simulink model "Baro"  (R2021a)
settings: Solver=VariableStepAuto  StartTime=0.0  StopTime=10.0  RelTol=1e-3
undefined symbols (not defined in the file or in its folder): Sensor_err
libraries: dspsrcs4 x1
settings Model: Creator=mojta  LastModifiedBy=mojta

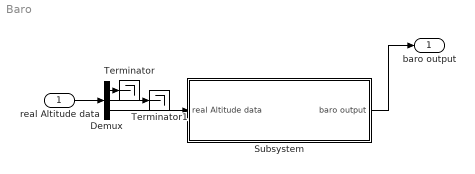
== system Baro ==
  real Altitude data : Inport
  Demux : Demux  Outputs=3
  Subsystem : Subsystem
  Terminator : Terminator
  Terminator1 : Terminator
  baro output : Outport
  wires:
  Demux/3 -> Subsystem/1(real Altitude data)
  Subsystem/1(baro output) -> baro output/1
  real Altitude data/1 -> Demux/1
  Demux/1 -> Terminator/1
  Demux/2 -> Terminator1/1

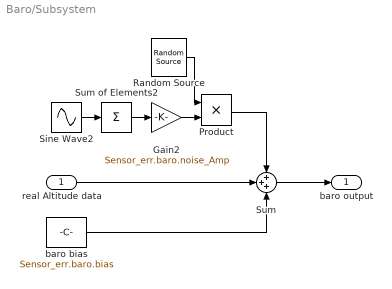
== system Baro/Subsystem ==
  real Altitude data : Inport
  Gain2 : Gain  Gain=Sensor_err.baro.noise_Amp
  Product : Product
  Random Source : dspsrcs4/Random Source  SrcType=Uniform  NormMethod=Ziggurat  CltLength=12  MinVal=0  MaxVal=1  MeanVal=0  VarVal=1  RepMode=Not repeatable  rawSeed=1  IsInherit=off  SampMode=Discrete  SampTime=1  SampFrame=1  DataType=Double  OutComplex=Real  OutputFrames=off
  Sine Wave2 : Sin  Frequency=2*pi*Sensor_err.baro.freqs  SampleTime=0
  Sum : Sum  Inputs=3
  Sum of Elements2 : Sum  Inputs=+
  baro bias : Constant  Value=Sensor_err.baro.bias
  baro output : Outport
  wires:
  Sum of Elements2/1 -> Gain2/1
  baro bias/1 -> Sum/3
  real Altitude data/1 -> Sum/2
  Sum/1 -> baro output/1
  Sine Wave2/1 -> Sum of Elements2/1
  Gain2/1 -> Product/2
  Random Source/1 -> Product/1
  Product/1 -> Sum/1
